simulink model "RunFMUfromMatlabFMU"  (R2023b)
settings: Solver=VariableStepAuto  StartTime=0.0  StopTime=50  RelTol=1e-3
values from neighbouring files (symbols this model uses):
  g = 9.8    [SetVehicleParameters.m]    (also in SetVehicleParameters2.m; SetVehicleParameters4.m; SetVehicleParameters5.m; SetVehicleParameters6.m)
  inSteering = .1    (= 0.1)    [RunFMUfromMatlab.m]
  inTorqueLeft = 10    [RunFMUfromMatlab.m]
  inTorqueRight = 10    [RunFMUfromMatlab.m]
settings Model: Creator=denoc  LastModifiedBy=eludg

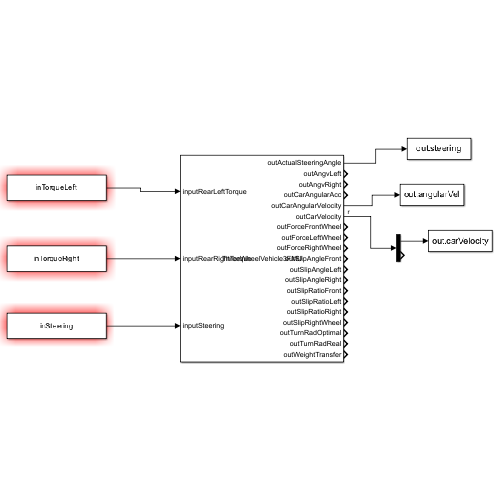
[thumbnail: Simulink's stored preview of the top-level diagram]
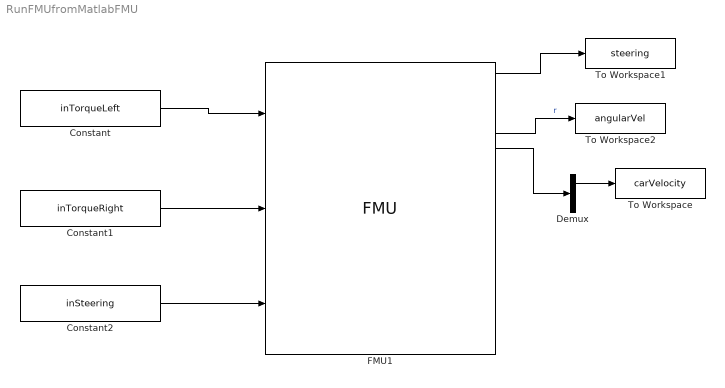
== system RunFMUfromMatlabFMU ==
  Constant : Constant  Value=inTorqueLeft
  Constant1 : Constant  Value=inTorqueRight
  Constant2 : Constant  Value=inSteering
  Demux : Demux  Outputs=2
  FMU1 : FMU  FMUName=ThreeWheelVehicle3FMUpid.fmu  FMUMode=ModelExchange  FMUInitializeEnumObject=off  FMUCachedDialogLayout="{\"Geometry\":[468,174,698,530],\"ParameterColumnsWidthConfig\":\"{\\\"columns\\\":[{\\\"name\\\":\\\"Parameter\\\",\\\"width\\\":550},{\\\"name\\\":\\\"Value\\\",\\\"width\\\":462},{\\\"name\\\":\\\"Unit\\\",\\\"width\\\":438},{\\\"name\\\":\\\"Description\\\",\\\"width\\\":571}]}\",\"InputColumnsWidthConfig\":[],\"OutputColumnsWidthConfig\":\"{\\\"columns\\\":[{\\\"name\\\":\\\"Name\\\",\\\"width\\\":558},{\\\"name\\\":\\\"Visibility\\\",\\\"width\\\":152},{\\\"name\\\":\\\"Start\\\",\\\"width\\\":266},{\\\"name\\\":\\\"Unit\\\",\\\"width\\\":260},{\\\"name\\\":\\\"Type Object\\\",\\\"width\\\":370}]}\"}"  airResistanceLongitudinal=struct('r',[0.0,1.0],'rho',1.18)  backLength=Lr  body2=struct('I',1e-08,'m',0.1)  c_rollF=rollResF  c_rollL=rollResL  c_rollR=rollResR  dragCoef=dragCoeff  front=struct('r',[0.0],'width',0.2)  front2=struct('r',[1e-10,0.0])  frontLength=Lf  frontTrail=struct('r',[0.0,-0.1])  frontWheel=struct('diameter',0.1,'r',[0.0,1.0],'v0_roll',0.1)  g=g  gearRatio=gearRatio  inertiaBody=Izz  inertiaWheelF=inertiaF  inertiaWheelL=inertiaL  inertiaWheelR=inertiaR  mass=mass  massCenterZ=h  muAF=muAF  muAL=muAL  muAR=muAR  muSF=muSF  muSL=muSL  muSR=muSR  neg=struct('k',-1.0)  neg2=struct('k',-1.0)  planarWorld=struct('constantGravity',[0.0,0.0],'defaultFrameDiameterFraction',40.0,'defaultN_to_m',1000.0,'defaultNm_to_m',1000.0,'defaultSpecularCoefficient',0.7,'defaultWidthFraction',20.0,'defaultZPosition',0.0,'gravityArrowTail',[0.0,0.0],'nominalLength',1.0)  positionPhi=struct('f_crit',50.0)  rear=struct('r',[0.0],'width',0.2)  rearLeft=struct('r',[0,0.0])  rearLeftWheel=struct('diameter',0.1,'r',[0.0,1.0],'v0_roll',0.1)  rearRight=struct('r',[0,0.0])  rearRightWheel=struct('diameter',0.1,'r',[0.0,1.0],'v0_roll',0.1)  sAdF=sAdF  sAdL=sAdL  sAdR=sAdR  sSlF=sSlF  sSlL=sSlL  sSlR=sSlR  speedStart=14  turnRadiusMAX=1000.0  vAdF=vAdF  vAdL=vAdL  vAdR=vAdR  vSlF=vSlF  vSlL=vSlL  vSlR=vSlR  vehicleFrontArea=1.5  vehicleWidth=rearTrackWidth  wheelRadiusF=wheelRadiusF  wheelRadiusL=wheelRadiusL  wheelRadiusR=wheelRadiusR  body_sphere_shapeType=sphere  body2_sphere_shapeType=sphere  front_cylinder_shapeType=cylinder  front2_cylinder_shapeType=cylinder  frontTrail_cylinder_shapeType=cylinder  frontWheel_cylinder_shapeType=cylinder  frontWheel_rim1_shapeType=cylinder  frontWheel_rim2_shapeType=cylinder  planarWorld_label1=x  planarWorld_label2=y  rear_cylinder_shapeType=cylinder  rearLeft_cylinder_shapeType=cylinder  rearLeftWheel_cylinder_shapeType=cylinder  rearLeftWheel_rim1_shapeType=cylinder  rearLeftWheel_rim2_shapeType=cylinder  rearRight_cylinder_shapeType=cylinder  rearRightWheel_cylinder_shapeType=cylinder  rearRightWheel_rim1_shapeType=cylinder  rearRightWheel_rim2_shapeType=cylinder  revolute_cylinder_shapeType=cylinder  mask(ThreeWheelVehicle3FMU [Model Exchange, v2.0]){}
      settings: MultithreadedSim=off
      mask Display:
      | disp('ThreeWheelVehicle3FMU');
      | port_label('output',1,'outActualSteeringAngle');
      | port_label('output',2,'outAngvLeft');
      | port_label('output',3,'outAngvRight');
      | port_label('output',4,'outCarAngularAcc');
      | port_label('output',5,'outCarAngularVelocity');
      | port_label('output',6,'outCarVelocity');
      | port_label('output',7,'outForceFrontWheel');
      | port_label('output',8,'outForceLeftWheel');
      | port_label('output',9,'outForceRightWheel');
      | port_label('output',10,'outSlipAngleFront');
      | port_label('output',11,'outSlipAngleLeft');
      | port_label('output',12,'outSlipAngleRight');
      | port_label('output',13,'outSlipRatioFront');
      | port_label('output',14,'outSlipRatioLeft');
      | port_label('output',15,'outSlipRatioRight');
      | port_label('output',16,'outSlipRightWheel');
      | port_label('output',17,'outTurnRadOptimal');
      | port_label('output',18,'outTurnRadReal');
      | port_label('output',19,'outWeightTransfer');
      | port_label('input',1,'inputRearLeftTorque');
      | port_label('input',2,'inputRearRightTorque');
      | port_label('input',3,'inputSteering');
  To Workspace : ToWorkspace  VariableName=carVelocity  SaveFormat=Timeseries  SampleTime=-1
  To Workspace1 : ToWorkspace  VariableName=steering  SaveFormat=Timeseries  SampleTime=-1
  To Workspace2 : ToWorkspace  VariableName=angularVel  SaveFormat=Timeseries  SampleTime=-1
  wires:
  Constant/1 -> FMU1/1
  Constant1/1 -> FMU1/2
  Constant2/1 -> FMU1/3
  FMU1/6 -> Demux/1
  Demux/1 -> To Workspace/1
  FMU1/1 -> To Workspace1/1
  FMU1/5 -> To Workspace2/1  "r"
